simulink model "lab10simb"  (R2020a)
settings: Solver=ode4  StartTime=0.0  StopTime=100  FixedStep=0.01  RelTol=1e-3
settings Model: Creator=ariana  LastModifiedBy=ariana

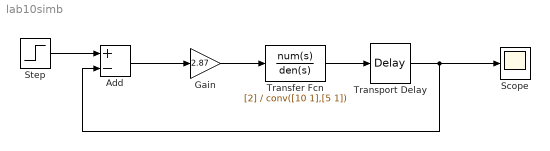
== system lab10simb ==
  Add : Sum  Inputs=+-
  Gain : Gain  Gain=2.87
  Scope : Scope
  Step : Step  Time=0  SampleTime=0
  Transfer Fcn : TransferFcn  Numerator=[2]  Denominator=conv([10 1],[5 1])
  Transport Delay : TransportDelay  DelayTime=3
  wires:
  Add/1 -> Gain/1
  Gain/1 -> Transfer Fcn/1
  Transfer Fcn/1 -> Transport Delay/1
  Step/1 -> Add/1
  Transport Delay/1 -> Add/2, Scope/1
